simulink subsystem "gqVector"  (R2024b)
settings: Solver=VariableStepAuto  StartTime=0.0  StopTime=10.0  RelTol=1e-3
values from neighbouring files (symbols this model uses):
  g = 9.81    [Plant_balrob_params.m]
undefined symbols (not defined in the file or in its folder): body, mot
settings Model: Creator=federico  LastModifiedBy=federico

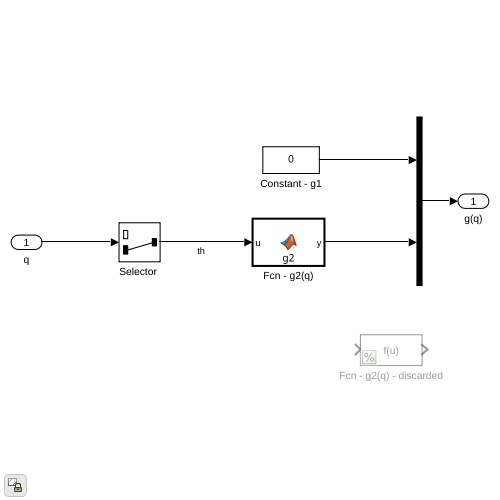
[thumbnail: Simulink's stored preview of the top-level diagram]
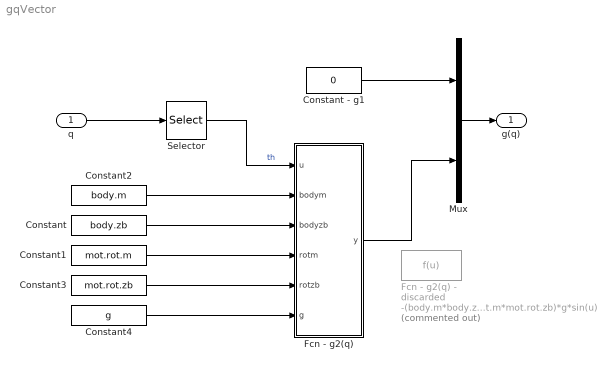
== system gqVector ==
  q : Inport
  Constant : Constant  Value=body.zb
  Constant - g1 : Constant  Value=0
  Constant1 : Constant  Value=mot.rot.m
  Constant2 : Constant  Value=body.m
  Constant3 : Constant  Value=mot.rot.zb
  Constant4 : Constant  Value=g
  Fcn - g2(q) : MATLAB Function  TreatAsAtomicUnit=on
  Fcn - g2(q) - discarded : Fcn  Commented=on  Expr=-(body.m*body.zb + 2*mot.rot.m*mot.rot.zb)*g*sin(u)
  Mux : Mux  Inputs=2
  "Selector " : Selector  InputPortWidth=2  IndexOptions=Index vector (dialog)  Indices=[2]  OutputSizes=1
  g(q) : Outport
  wires:
  Mux/1 -> g(q)/1
  Constant - g1/1 -> Mux/1
  Fcn - g2(q)/1(y) -> Mux/2
  "Selector "/1 -> Fcn - g2(q)/1(u)  "th"
  q/1 -> "Selector "/1
  Constant4/1 -> Fcn - g2(q)/6(g)
  Constant3/1 -> Fcn - g2(q)/5(rotzb)
  Constant1/1 -> Fcn - g2(q)/4(rotm)
  Constant/1 -> Fcn - g2(q)/3(bodyzb)
  Constant2/1 -> Fcn - g2(q)/2(bodym)

== matlab function gqVector/Fcn - g2(q) ==
  data: u input; y output; bodym input; bodyzb input; rotm input; rotzb input; g input
function y = g2(u, bodym, bodyzb, rotm, rotzb, g)

y = -(bodym*bodyzb + 2*rotm*rotzb)*g*sin(u);
